simulink model "planRoute_sim"  (R2024a)
settings: Solver=FixedStepDiscrete  StartTime=0.0  StopTime=0  RelTol=1e-3
InitFcn:
  | routePlanSetup
undefined symbols (not defined in the file): goal, gridLoc, pathBus_struct, res, start, tuneableTerrainAwareParams, worldMat
libraries: roshelperlib x2
settings Model: Creator=cstabile  LastModifiedBy=cstabile

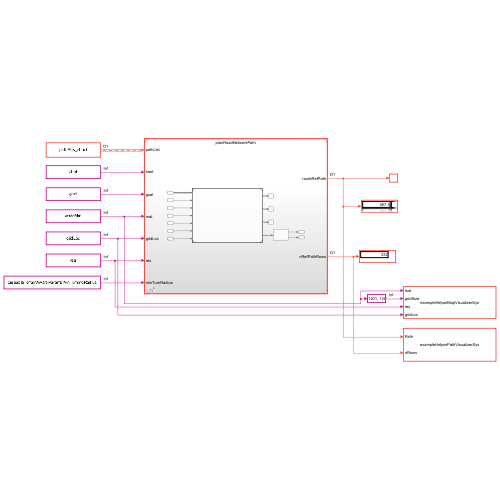
[thumbnail: Simulink's stored preview of the top-level diagram]
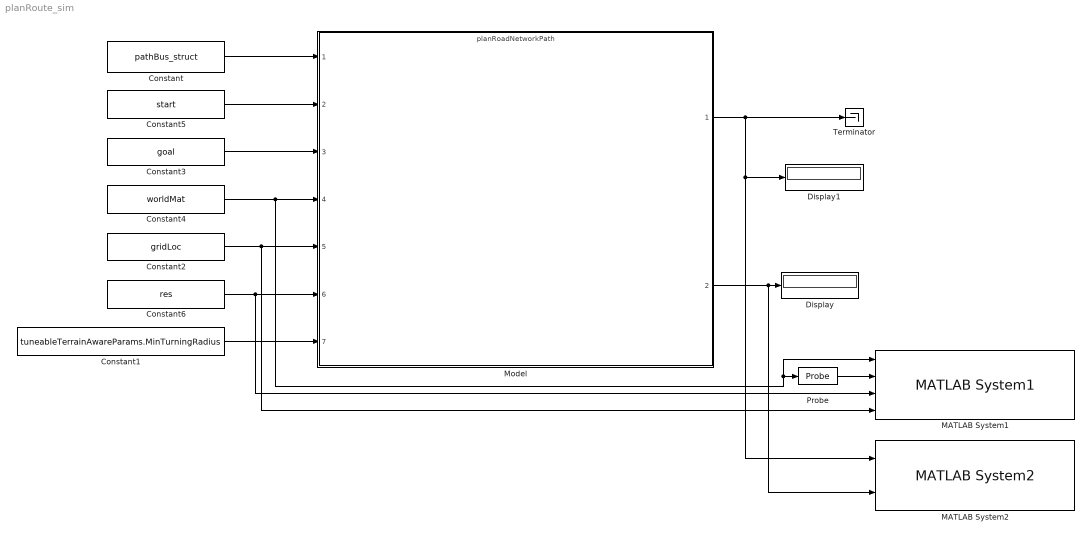
== system planRoute_sim ==
  Constant : Constant  Value=pathBus_struct  VectorParams1D=off  OutDataTypeStr=Bus: pathList_fixed_bus  SampleTime=-1
  Constant1 : Constant  Value=tuneableTerrainAwareParams.MinTurningRadius
  Constant2 : Constant  Value=gridLoc
  Constant3 : Constant  Value=goal
  Constant4 : Constant  Value=worldMat
  Constant5 : Constant  Value=start
  Constant6 : Constant  Value=res
  Display : Display
  Display1 : Display
  MATLAB System1 : roshelperlib/MATLAB System1  MapType=SDF  DisplayVisual=on  SimulateUsing=Interpreted execution
  MATLAB System2 : roshelperlib/MATLAB System2  VisualizationParameters={'k-'}  PlotType=Line  DisplayVisual=on  SimulateUsing=Interpreted execution
  Model : ModelReference  ModelNameDialog=planRoadNetworkPath.slx  SimulationMode=Normal  ModelReferenceVersion=1.0
  Probe : Probe  ProbeWidth=off  ProbeSampleTime=off  ProbeComplexSignal=off  ProbeSignalDimensions=on
  Terminator : Terminator
  wires:
  Constant5/1 -> Model/2
  Constant3/1 -> Model/3
  Constant4/1 -> MATLAB System1/1, Probe/1, Model/4
  Constant2/1 -> MATLAB System1/4, Model/5
  Constant6/1 -> MATLAB System1/3, Model/6
  Constant1/1 -> Model/7
  Model/1 -> MATLAB System2/1, Display1/1, Terminator/1
  Model/2 -> MATLAB System2/2, Display/1
  Probe/1 -> MATLAB System1/2
  Constant/1 -> Model/1
